simulink model "Energy_Cost"  (Simulink 8.8)
settings: Solver=ode23t  StartTime=0.0  StopTime=24  RelTol=1e-3  EnableMultiTasking=on
model workspace: external: MAT-File (data not in the file)
libraries: simulink x4
(part 4 of 5)

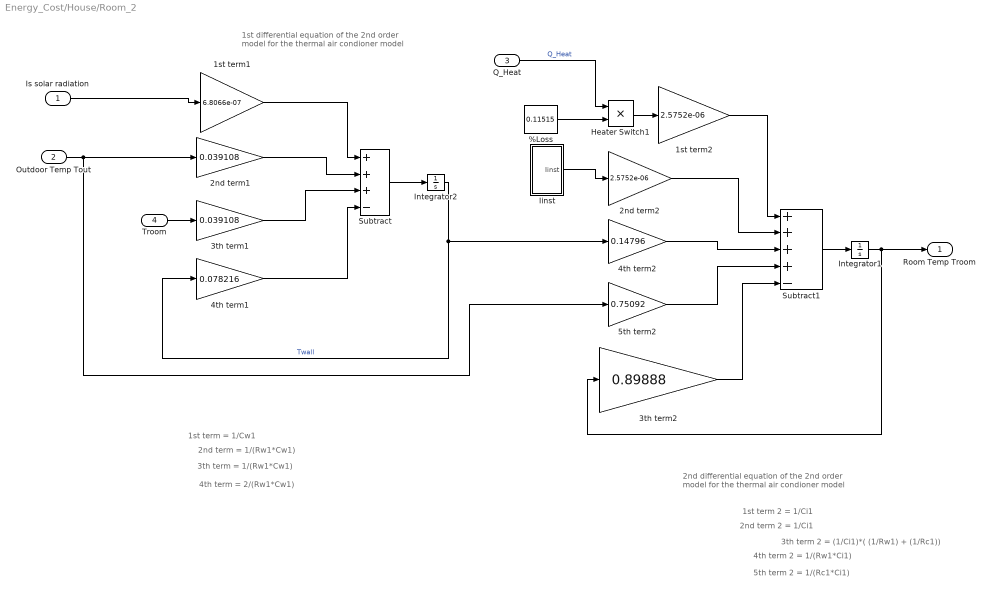
== system Energy_Cost/House/Room_2 ==
  note: 1st differential equation of the 2nd order
      | model for the thermal air condioner model
  note: 2nd differential equation of the 2nd order
      | model for the thermal air condioner model
  note: 1st term = 1/Cw1
  note: 2nd term = 1/(Rw1*Cw1)
  note: 3th term = 1/(Rw1*Cw1)
  note: 4th term = 2/(Rw1*Cw1)
  note: 1st term 2 = 1/Ci1
  note: 2nd term 2 = 1/Ci1
  note: 3th term 2 = (1/Ci1)*( (1/Rw1) + (1/Rc1))
  note: 4th term 2 = 1/(Rw1*Ci1)
  note: 5th term 2 = 1/(Rc1*Ci1)
  Is solar radiation : Inport
  Outdoor Temp Tout : Inport  Port=2
  Q_Heat : Inport  Port=3
  Troom : Inport  Port=4
  %Loss : Constant  Value=0.11515
  1st term1 : Gain  Gain=6.8066e-07
  1st term2 : Gain  Gain=2.5752e-06
  2nd term1 : Gain  Gain=0.039108
  2nd term2 : Gain  Gain=2.5752e-06
  3th term1 : Gain  Gain=0.039108
  3th term2 : Gain  Gain=0.89888
  4th term1 : Gain  Gain=0.078216
  4th term2 : Gain  Gain=0.14796
  5th term2 : Gain  Gain=0.75092
  Heater Switch1 : Product  RndMeth=Zero
  Iinst : Subsystem
  Integrator1 : Integrator  InitialCondition=21
  Integrator2 : Integrator  InitialCondition=21
  Subtract : Sum  Inputs=+++-
  Subtract1 : Sum  Inputs=++++-
  Room Temp Troom : Outport  InitialOutput=0
  wires:
  2nd term1/1 -> Subtract/2
  4th term1/1 -> Subtract/4
  Subtract/1 -> Integrator2/1
  Integrator2/1 -> 4th term1/1, 4th term2/1  "Twall"
  Integrator1/1 -> 3th term2/1, Room Temp Troom/1
  Subtract1/1 -> Integrator1/1
  Outdoor Temp Tout/1 -> 2nd term1/1, 5th term2/1
  Troom/1 -> 3th term1/1
  3th term1/1 -> Subtract/3
  1st term1/1 -> Subtract/1
  2nd term2/1 -> Subtract1/2
  Q_Heat/1 -> Heater Switch1/1  "Q_Heat"
  Iinst/1(Iinst) -> 2nd term2/1
  Is solar radiation/1 -> 1st term1/1
  4th term2/1 -> Subtract1/3
  5th term2/1 -> Subtract1/4
  3th term2/1 -> Subtract1/5
  %Loss/1 -> Heater Switch1/2
  Heater Switch1/1 -> 1st term2/1
  1st term2/1 -> Subtract1/1

== system Energy_Cost/House/Room_3 ==
  note: 1st differential equation of the 2nd order
      | model for the thermal air condioner model
  note: 2nd differential equation of the 2nd order
      | model for the thermal air condioner model
  note: 1st term = 1/Cw1
  note: 2nd term = 1/(Rw1*Cw1)
  note: 3th term = 1/(Rw1*Cw1)
  note: 4th term = 2/(Rw1*Cw1)
  note: 1st term 2 = 1/Ci1
  note: 2nd term 2 = 1/Ci1
  note: 3th term 2 = (1/Ci1)*( (1/Rw1) + (1/Rc1))
  note: 4th term 2 = 1/(Rw1*Ci1)
  note: 5th term 2 = 1/(Rc1*Ci1)
  Is solar radiation : Inport
  Outdoor Temp Tout : Inport  Port=2
  Q_Heat : Inport  Port=3
  Troom : Inport  Port=4
  %Loss : Constant  Value=0.11638
  1st term1 : Gain  Gain=6.0825e-07
  1st term2 : Gain  Gain=2.2533e-06
  2nd term1 : Gain  Gain=0.039108
  2nd term2 : Gain  Gain=2.2533e-06
  3th term1 : Gain  Gain=0.039108
  3th term2 : Gain  Gain=0.80194
  4th term1 : Gain  Gain=0.078216
  4th term2 : Gain  Gain=0.14488
  5th term2 : Gain  Gain=0.65706
  Heater Switch1 : Product  RndMeth=Zero
  Iinst : Subsystem
  Integrator1 : Integrator  InitialCondition=21
  Integrator2 : Integrator  InitialCondition=21
  Subtract : Sum  Inputs=+++-
  Subtract1 : Sum  Inputs=++++-
  Room Temp Troom : Outport  InitialOutput=0
  wires:
  2nd term1/1 -> Subtract/2
  4th term1/1 -> Subtract/4
  Subtract/1 -> Integrator2/1
  Integrator2/1 -> 4th term1/1, 4th term2/1  "Twall"
  Integrator1/1 -> 3th term2/1, Room Temp Troom/1
  Subtract1/1 -> Integrator1/1
  Outdoor Temp Tout/1 -> 2nd term1/1, 5th term2/1
  Troom/1 -> 3th term1/1
  3th term1/1 -> Subtract/3
  1st term1/1 -> Subtract/1
  2nd term2/1 -> Subtract1/2
  Q_Heat/1 -> Heater Switch1/1  "Q_Heat"
  Iinst/1(Iinst) -> 2nd term2/1
  Is solar radiation/1 -> 1st term1/1
  4th term2/1 -> Subtract1/3
  5th term2/1 -> Subtract1/4
  3th term2/1 -> Subtract1/5
  %Loss/1 -> Heater Switch1/2
  1st term2/1 -> Subtract1/1
  Heater Switch1/1 -> 1st term2/1

== system Energy_Cost/House/Room_4 ==
  note: 1st differential equation of the 2nd order
      | model for the thermal air condioner model
  note: 2nd differential equation of the 2nd order
      | model for the thermal air condioner model
  note: 1st term = 1/Cw1
  note: 2nd term = 1/(Rw1*Cw1)
  note: 3th term = 1/(Rw1*Cw1)
  note: 4th term = 2/(Rw1*Cw1)
  note: 1st term 2 = 1/Ci1
  note: 2nd term 2 = 1/Ci1
  note: 3th term 2 = (1/Ci1)*( (1/Rw1) + (1/Rc1))
  note: 4th term 2 = 1/(Rw1*Ci1)
  note: 5th term 2 = 1/(Rc1*Ci1)
  Is solar radiation : Inport
  Outdoor Temp Tout : Inport  Port=2
  Q_Heat : Inport  Port=3
  Troom : Inport  Port=4
  %Loss : Constant  Value=0.11393
  1st term1 : Gain  Gain=7.7264e-07
  1st term2 : Gain  Gain=3.0044e-06
  2nd term1 : Gain  Gain=0.039108
  2nd term2 : Gain  Gain=3.0044e-06
  3th term1 : Gain  Gain=0.039108
  3th term2 : Gain  Gain=1.0281
  4th term1 : Gain  Gain=0.078216
  4th term2 : Gain  Gain=0.15207
  5th term2 : Gain  Gain=0.87608
  Heater Switch1 : Product  RndMeth=Zero
  Iinst : Subsystem
  Integrator1 : Integrator  InitialCondition=21
  Integrator2 : Integrator  InitialCondition=21
  Subtract : Sum  Inputs=+++-
  Subtract1 : Sum  Inputs=++++-
  Room Temp Troom : Outport  InitialOutput=0
  wires:
  2nd term1/1 -> Subtract/2
  4th term1/1 -> Subtract/4
  Subtract/1 -> Integrator2/1
  Integrator2/1 -> 4th term1/1, 4th term2/1  "Twall"
  Integrator1/1 -> 3th term2/1, Room Temp Troom/1
  Subtract1/1 -> Integrator1/1
  Outdoor Temp Tout/1 -> 2nd term1/1, 5th term2/1
  Troom/1 -> 3th term1/1
  3th term1/1 -> Subtract/3
  1st term1/1 -> Subtract/1
  2nd term2/1 -> Subtract1/2
  Q_Heat/1 -> Heater Switch1/1  "Q_Heat"
  Iinst/1(Iinst) -> 2nd term2/1
  Is solar radiation/1 -> 1st term1/1
  4th term2/1 -> Subtract1/3
  5th term2/1 -> Subtract1/4
  3th term2/1 -> Subtract1/5
  %Loss/1 -> Heater Switch1/2
  Heater Switch1/1 -> 1st term2/1
  1st term2/1 -> Subtract1/1

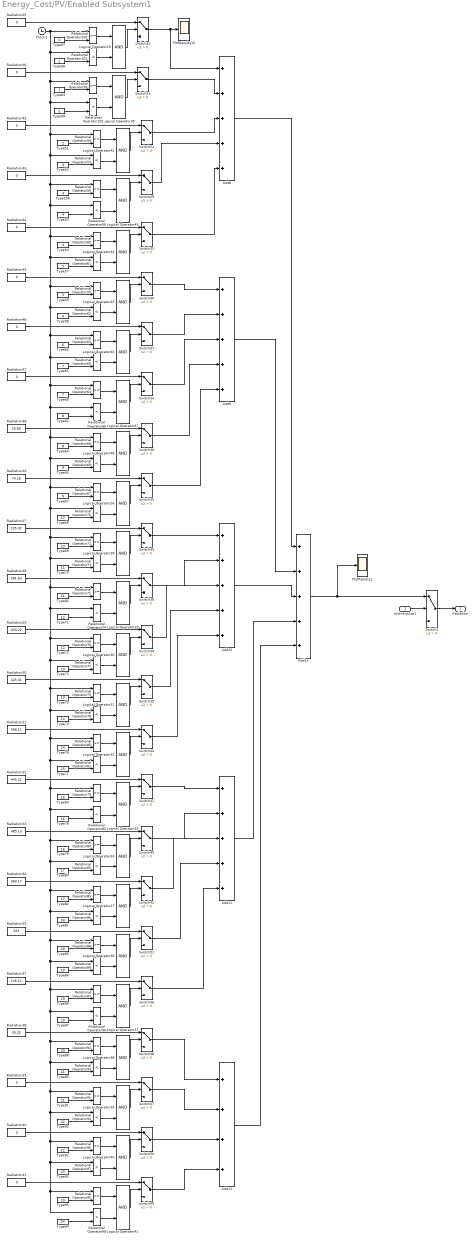
== system Energy_Cost/PV/Enabled Subsystem1 ==
  active pulse1 : Inport
  Add{8..11,13} (5 alike) : Sum  Inputs=+++++
  Add12 : Sum  Inputs=++++
  Clock2 : Clock
  Logical Operator{19,26..48} (24 alike) : Logic  AllPortsSameDT=off  OutDataTypeStr=boolean
  PlotResults1 : Scope
  PlotResults10 : Scope
  Radiation{25,36,39..47} (11 alike) : Constant  Value=0
  Radiation26 : Constant  Value=74.18
  Radiation27 : Constant  Value=195.32
  Radiation28 : Constant  Value=281.63
  Radiation29 : Constant  Value=453.22
  Radiation30 : Constant  Value=425.31
  Radiation31 : Constant  Value=556.11
  Radiation32 : Constant  Value=445.22
  Radiation33 : Constant  Value=485.13
  Radiation34 : Constant  Value=360.17
  Radiation35 : Constant  Value=253
  Radiation37 : Constant  Value=126.11
  Radiation38 : Constant  Value=33.25
  Radiation48 : Constant  Value=25.85
  Relational Operator{55..56,59..60,63..64,67..68,71..72,75..76,79..80,83..84,87..88,91..92,95..96,99..100} (24 alike) : RelationalOperator  RndMeth=Nearest  InputSameDT=on
  Relational Operator{57..58,61..62,65..66,69..70,73..74,77..78,81..82,85..86,89..90,93..94,97..98,101..102} (24 alike) : RelationalOperator  Operator=<  RndMeth=Nearest  InputSameDT=on
  Switch{1,29..30,33..54} (25 alike) : Switch  Criteria=u2 > Threshold
  Type100 : Constant  Value=3
  Type51 : Constant  Value=2
  Type52 : Constant  Value=3
  Type53 : Constant  Value=4
  Type54 : Constant  Value=4
  Type57 : Constant  Value=5
  Type58 : Constant  Value=6
  Type59 : Constant  Value=5
  Type60 : Constant  Value=6
  Type61 : Constant  Value=7
  Type62 : Constant  Value=8
  Type63 : Constant
  Type64 : Constant  Value=8
  Type65 : Constant  Value=9
  Type66 : Constant  Value=10
  Type67 : Constant  Value=9
  Type68 : Constant  Value=7
  Type69 : Constant  Value=10
  Type70 : Constant  Value=11
  Type71 : Constant  Value=12
  Type72 : Constant  Value=12
  Type73 : Constant  Value=13
  Type74 : Constant  Value=14
  Type75 : Constant  Value=13
  Type76 : Constant  Value=14
  Type77 : Constant  Value=15
  Type78 : Constant  Value=16
  Type79 : Constant  Value=16
  Type80 : Constant  Value=17
  Type81 : Constant  Value=18
  Type82 : Constant  Value=17
  Type83 : Constant  Value=15
  Type84 : Constant  Value=11
  Type85 : Constant  Value=18
  Type86 : Constant  Value=19
  Type87 : Constant  Value=20
  Type88 : Constant  Value=20
  Type89 : Constant  Value=21
  Type90 : Constant  Value=22
  Type91 : Constant  Value=21
  Type92 : Constant  Value=22
  Type93 : Constant  Value=23
  Type94 : Constant  Value=24
  Type95 : Constant  Value=23
  Type96 : Constant  Value=19
  Type97 : Constant  Value=0
  Type98 : Constant
  Type99 : Constant  Value=2
  Radiation : Outport
  wires:
  Switch1/1 -> Radiation/1
  active pulse1/1 -> Switch1/2
  Radiation25/1 -> Switch52/1
  Switch52/1 -> PlotResults10/1, Add8/1
  Clock2/1 -> Relational Operator100/1, Relational Operator101/1, Relational Operator99/1, Relational Operator102/1, Relational Operator64/1, Relational Operator65/1, Relational Operator63/1, Relational Operator66/1, Relational Operator68/1, Relational Operator69/1, Relational Operator67/1, Relational Operator70/1, Relational Operator72/1, Relational Operator73/1, Relational Operator71/1, Relational Operator76/1, Relational Operator75/1, Relational Operator78/1, Relational Operator80/1, Relational Operator81/1, Relational Operator79/1, Relational Operator82/1, Relational Operator84/1, Relational Operator85/1, Relational Operator83/1, Relational Operator86/1, Relational Operator89/1, Relational Operator87/1, Relational Operator91/1, Relational Operator98/1, Relational Operator95/1, Relational Operator97/1, Relational Operator96/1, Relational Operator94/1, Relational Operator93/1, Relational Operator92/1, Relational Operator90/1, Relational Operator88/1, Relational Operator77/1, Relational Operator74/1, Relational Operator62/1, Relational Operator59/1, Relational Operator61/1, Relational Operator60/1, Relational Operator58/1, Relational Operator55/1, Relational Operator57/1, Relational Operator56/1
  Type97/1 -> Relational Operator100/2
  Type98/1 -> Relational Operator101/2
  Relational Operator101/1 -> Logical Operator19/2
  Relational Operator100/1 -> Logical Operator19/1
  Logical Operator19/1 -> Switch52/2
  Radiation36/1 -> Switch53/1
  Type63/1 -> Relational Operator99/2
  Type99/1 -> Relational Operator102/2
  Relational Operator102/1 -> Logical Operator35/2
  Relational Operator99/1 -> Logical Operator35/1
  Logical Operator35/1 -> Switch53/2
  Type51/1 -> Relational Operator56/2
  Type52/1 -> Relational Operator57/2
  Relational Operator57/1 -> Logical Operator42/2
  Relational Operator56/1 -> Logical Operator42/1
  Logical Operator42/1 -> Switch54/2
  Type100/1 -> Relational Operator55/2
  Type53/1 -> Relational Operator58/2
  Relational Operator58/1 -> Logical Operator43/2
  Relational Operator55/1 -> Logical Operator43/1
  Logical Operator43/1 -> Switch29/2
  Type54/1 -> Relational Operator60/2
  Type57/1 -> Relational Operator61/2
  Relational Operator61/1 -> Logical Operator44/2
  Relational Operator60/1 -> Logical Operator44/1
  Logical Operator44/1 -> Switch33/2
  Type59/1 -> Relational Operator59/2
  Type58/1 -> Relational Operator62/2
  Relational Operator62/1 -> Logical Operator45/2
  Relational Operator59/1 -> Logical Operator45/1
  Logical Operator45/1 -> Switch30/2
  Type60/1 -> Relational Operator64/2
  Type61/1 -> Relational Operator65/2
  Relational Operator65/1 -> Logical Operator46/2
  Relational Operator64/1 -> Logical Operator46/1
  Logical Operator46/1 -> Switch37/2
  Type68/1 -> Relational Operator63/2
  Type62/1 -> Relational Operator66/2
  Relational Operator66/1 -> Logical Operator47/2
  Relational Operator63/1 -> Logical Operator47/1
  Logical Operator47/1 -> Switch34/2
  Type64/1 -> Relational Operator68/2
  Type65/1 -> Relational Operator69/2
  Relational Operator69/1 -> Logical Operator48/2
  Relational Operator68/1 -> Logical Operator48/1
  Logical Operator48/1 -> Switch36/2
  Type67/1 -> Relational Operator67/2
  Type66/1 -> Relational Operator70/2
  Relational Operator70/1 -> Logical Operator26/2
  Relational Operator67/1 -> Logical Operator26/1
  Logical Operator26/1 -> Switch35/2
  Type69/1 -> Relational Operator72/2
  Type70/1 -> Relational Operator73/2
  Relational Operator73/1 -> Logical Operator28/2
  Relational Operator72/1 -> Logical Operator28/1
  Logical Operator28/1 -> Switch45/2
  Type84/1 -> Relational Operator71/2
  Type71/1 -> Relational Operator74/2
  Relational Operator74/1 -> Logical Operator29/2
  Relational Operator71/1 -> Logical Operator29/1
  Logical Operator29/1 -> Switch38/2
  Type72/1 -> Relational Operator76/2
  Type73/1 -> Relational Operator77/2
  Relational Operator77/1 -> Logical Operator30/2
  Relational Operator76/1 -> Logical Operator30/1
  Logical Operator30/1 -> Switch40/2
  Type75/1 -> Relational Operator75/2
  Type74/1 -> Relational Operator78/2
  Relational Operator78/1 -> Logical Operator31/2
  Relational Operator75/1 -> Logical Operator31/1
  Logical Operator31/1 -> Switch39/2
  Type76/1 -> Relational Operator80/2
  Type77/1 -> Relational Operator81/2
  Relational Operator81/1 -> Logical Operator32/2
  Relational Operator80/1 -> Logical Operator32/1
  Logical Operator32/1 -> Switch44/2
  Type83/1 -> Relational Operator79/2
  Type78/1 -> Relational Operator82/2
  Relational Operator82/1 -> Logical Operator33/2
  Relational Operator79/1 -> Logical Operator33/1
  Logical Operator33/1 -> Switch41/2
  Type79/1 -> Relational Operator84/2
  Type80/1 -> Relational Operator85/2
  Relational Operator85/1 -> Logical Operator34/2
  Relational Operator84/1 -> Logical Operator34/1
  Logical Operator34/1 -> Switch43/2
  Type82/1 -> Relational Operator83/2
  Type81/1 -> Relational Operator86/2
  Relational Operator86/1 -> Logical Operator27/2
  Relational Operator83/1 -> Logical Operator27/1
  Logical Operator27/1 -> Switch42/2
  Type85/1 -> Relational Operator88/2
  Type86/1 -> Relational Operator89/2
  Relational Operator89/1 -> Logical Operator36/2
  Relational Operator88/1 -> Logical Operator36/1
  Logical Operator36/1 -> Switch51/2
  Type96/1 -> Relational Operator87/2
  Type87/1 -> Relational Operator90/2
  Relational Operator90/1 -> Logical Operator37/2
  Relational Operator87/1 -> Logical Operator37/1
  Logical Operator37/1 -> Switch46/2
  Type88/1 -> Relational Operator92/2
  Type89/1 -> Relational Operator93/2
  Relational Operator93/1 -> Logical Operator38/2
  Relational Operator92/1 -> Logical Operator38/1
  Logical Operator38/1 -> Switch48/2
  Type91/1 -> Relational Operator91/2
  Type90/1 -> Relational Operator94/2
  Relational Operator94/1 -> Logical Operator39/2
  Relational Operator91/1 -> Logical Operator39/1
  Logical Operator39/1 -> Switch47/2
  Type92/1 -> Relational Operator96/2
  Type93/1 -> Relational Operator97/2
  Relational Operator97/1 -> Logical Operator40/2
  Relational Operator96/1 -> Logical Operator40/1
  Logical Operator40/1 -> Switch50/2
  Type95/1 -> Relational Operator95/2
  Type94/1 -> Relational Operator98/2
  Relational Operator98/1 -> Logical Operator41/2
  Relational Operator95/1 -> Logical Operator41/1
  Logical Operator41/1 -> Switch49/2
  Radiation42/1 -> Switch54/1
  Radiation43/1 -> Switch29/1
  Radiation44/1 -> Switch33/1
  Radiation45/1 -> Switch30/1
  Radiation46/1 -> Switch37/1
  Radiation47/1 -> Switch34/1
  Radiation48/1 -> Switch36/1
  Radiation26/1 -> Switch35/1
  Radiation27/1 -> Switch45/1
  Radiation28/1 -> Switch38/1
  Radiation29/1 -> Switch40/1
  Radiation30/1 -> Switch39/1
  Radiation31/1 -> Switch44/1
  Radiation32/1 -> Switch41/1
  Radiation33/1 -> Switch43/1
  Radiation34/1 -> Switch42/1
  Radiation35/1 -> Switch51/1
  Radiation37/1 -> Switch46/1
  Radiation38/1 -> Switch48/1
  Radiation39/1 -> Switch47/1
  Radiation40/1 -> Switch50/1
  Radiation41/1 -> Switch49/1
  Switch53/1 -> Add8/2
  Switch54/1 -> Add8/3
  Switch33/1 -> Add8/5
  Switch29/1 -> Add8/4
  Switch30/1 -> Add9/1
  Switch37/1 -> Add9/2
  Switch34/1 -> Add9/3
  Switch36/1 -> Add9/4
  Switch35/1 -> Add9/5
  Switch45/1 -> Add10/1
  Switch38/1 -> Add10/2
  Switch40/1 -> Add10/3
  Switch39/1 -> Add10/4
  Switch44/1 -> Add10/5
  Switch41/1 -> Add11/1
  Switch43/1 -> Add11/2
  Switch42/1 -> Add11/3
  Switch51/1 -> Add11/4
  Switch46/1 -> Add11/5
  Switch48/1 -> Add12/1
  Switch47/1 -> Add12/2
  Switch50/1 -> Add12/3
  Switch49/1 -> Add12/4
  Add8/1 -> Add13/1
  Add9/1 -> Add13/2
  Add10/1 -> Add13/3
  Add11/1 -> Add13/4
  Add12/1 -> Add13/5
  Add13/1 -> Switch1/1, PlotResults1/1

== system Energy_Cost/PV/Rates ==
  Powe_cons : Inport
  Rate_season2 : Inport  Port=2
  Clock1 : Clock
      settings: Decimation=100
  Constant : Constant  Value=6.2
  Constant1 : Constant  Value=10.8
  Constant2 : Constant  Value=9.2
  Electricity Rate : M-S-Function  FunctionName=Elec_Rate_Fun
  Heater Switch1 : Product  RndMeth=Zero
  Rate : Outport  InitialOutput=0
  wires:
  Powe_cons/1 -> Heater Switch1/2
  Heater Switch1/1 -> Rate/1
  Constant/1 -> Electricity Rate/1
  Clock1/1 -> Electricity Rate/4
  Rate_season2/1 -> Electricity Rate/5
  Electricity Rate/1 -> Heater Switch1/1  "Elec_Rate"
  Constant2/1 -> Electricity Rate/2
  Constant1/1 -> Electricity Rate/3

== system Energy_Cost/Refrigerator/Rates ==
  Powe_cons : Inport
  Rate_season2 : Inport  Port=2
  Clock2 : Clock
      settings: Decimation=100
  Ele_mid : Constant  Value=9.2
  Ele_off : Constant  Value=6.2
  Ele_peak : Constant  Value=10.8
  Electricity Rate : M-S-Function  FunctionName=Elec_Rate_Fun
  Heater Switch6 : Product  Inputs=3  RndMeth=Zero
  Rate_Ele_WH : Constant
  Rate : Outport  InitialOutput=0
  wires:
  Ele_off/1 -> Electricity Rate/1
  Ele_mid/1 -> Electricity Rate/2
  Ele_peak/1 -> Electricity Rate/3
  Clock2/1 -> Electricity Rate/4
  Rate_Ele_WH/1 -> Heater Switch6/1
  Heater Switch6/1 -> Rate/1
  Powe_cons/1 -> Heater Switch6/3
  Rate_season2/1 -> Electricity Rate/5
  Electricity Rate/1 -> Heater Switch6/2

== system Energy_Cost/Thermostat/If Action Subsystem ==
  In1 : Inport
  Action Port : ActionPort  ActionType=then
  Out1 : Outport
  wires:
  In1/1 -> Out1/1

== system Energy_Cost/Thermostat/If Action Subsystem1 ==
  In1 : Inport
  Action Port : ActionPort  ActionType=else
  Out1 : Outport
  wires:
  In1/1 -> Out1/1

== system Energy_Cost/Water Heater/Rates ==
  Powe_cons : Inport
  Clock2 : Clock
      settings: Decimation=100
  Constant : Constant
  Ele_mid : Constant  Value=9.2
  Ele_off : Constant  Value=6.2
  Ele_peak : Constant  Value=10.8
  Electricity Rate : M-S-Function  FunctionName=Elec_Rate_Fun
  Gas rate : Constant  Value=35.7
  Heater Switch2 : Product  Inputs=3  RndMeth=Zero
  Heater Switch6 : Product  Inputs=3  RndMeth=Zero
  Rate_Ele_WH : Constant  Value=0
  Rate_Gas_WH : Constant
  Rate_season : Constant
  Sum2 : Sum  SaturateOnIntegerOverflow=on  InputSameDT=on  OutDataTypeStr=Inherit: Same as first input
  c3=Watts/Pc : Gain  Gain=1/9.932  SaturateOnIntegerOverflow=on  OutDataTypeStr=Inherit: Same as input  ParamDataTypeStr=Inherit: Same as input
  Rate : Outport  InitialOutput=0
  Rate_season1 : Outport  Port=2  InitialOutput=0
  wires:
  Ele_off/1 -> Electricity Rate/1
  Ele_mid/1 -> Electricity Rate/2
  Ele_peak/1 -> Electricity Rate/3
  Clock2/1 -> Electricity Rate/4
  Rate_season/1 -> Electricity Rate/5, Rate_season1/1
  Rate_Ele_WH/1 -> Heater Switch6/1
  Powe_cons/1 -> c3=Watts/Pc/1, Heater Switch6/3
  c3=Watts/Pc/1 -> Heater Switch2/1
  Gas rate/1 -> Heater Switch2/2
  Rate_Gas_WH/1 -> Heater Switch2/3
  Heater Switch6/1 -> Sum2/1
  Heater Switch2/1 -> Sum2/2
  Sum2/1 -> Rate/1
  Electricity Rate/1 -> Heater Switch6/2

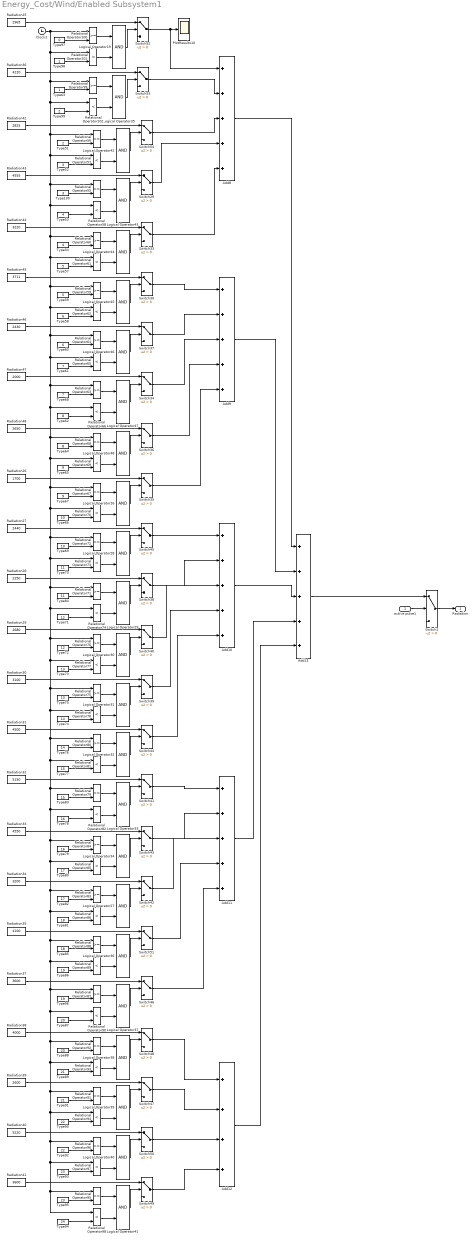
== system Energy_Cost/Wind/Enabled Subsystem1 ==
  active pulse1 : Inport
  Add{8..11,13} (5 alike) : Sum  Inputs=+++++
  Add12 : Sum  Inputs=++++
  Clock2 : Clock
  Logical Operator{19,26..48} (24 alike) : Logic  AllPortsSameDT=off  OutDataTypeStr=boolean
  PlotResults10 : Scope
  Radiation25 : Constant  Value=2965
  Radiation26 : Constant  Value=1700
  Radiation27 : Constant  Value=2440
  Radiation28 : Constant  Value=2250
  Radiation29 : Constant  Value=2680
  Radiation30 : Constant  Value=3100
  Radiation31 : Constant  Value=4500
  Radiation32 : Constant  Value=5150
  Radiation33 : Constant  Value=4550
  Radiation34 : Constant  Value=3200
  Radiation35 : Constant  Value=4100
  Radiation36 : Constant  Value=4220
  Radiation37 : Constant  Value=3600
  Radiation38 : Constant  Value=4000
  Radiation39 : Constant  Value=2600
  Radiation40 : Constant  Value=5220
  Radiation41 : Constant  Value=3600
  Radiation42 : Constant  Value=2825
  Radiation43 : Constant  Value=4555
  Radiation44 : Constant  Value=3220
  Radiation45 : Constant  Value=3711
  Radiation46 : Constant  Value=2430
  Radiation47 : Constant  Value=2000
  Radiation48 : Constant  Value=2650
  Relational Operator{55..56,59..60,63..64,67..68,71..72,75..76,79..80,83..84,87..88,91..92,95..96,99..100} (24 alike) : RelationalOperator  RndMeth=Nearest  InputSameDT=on
  Relational Operator{57..58,61..62,65..66,69..70,73..74,77..78,81..82,85..86,89..90,93..94,97..98,101..102} (24 alike) : RelationalOperator  Operator=<  RndMeth=Nearest  InputSameDT=on
  Switch{1,29..30,33..54} (25 alike) : Switch  Criteria=u2 > Threshold
  Type100 : Constant  Value=3
  Type51 : Constant  Value=2
  Type52 : Constant  Value=3
  Type53 : Constant  Value=4
  Type54 : Constant  Value=4
  Type57 : Constant  Value=5
  Type58 : Constant  Value=6
  Type59 : Constant  Value=5
  Type60 : Constant  Value=6
  Type61 : Constant  Value=7
  Type62 : Constant  Value=8
  Type63 : Constant
  Type64 : Constant  Value=8
  Type65 : Constant  Value=9
  Type66 : Constant  Value=10
  Type67 : Constant  Value=9
  Type68 : Constant  Value=7
  Type69 : Constant  Value=10
  Type70 : Constant  Value=11
  Type71 : Constant  Value=12
  Type72 : Constant  Value=12
  Type73 : Constant  Value=13
  Type74 : Constant  Value=14
  Type75 : Constant  Value=13
  Type76 : Constant  Value=14
  Type77 : Constant  Value=15
  Type78 : Constant  Value=16
  Type79 : Constant  Value=16
  Type80 : Constant  Value=17
  Type81 : Constant  Value=18
  Type82 : Constant  Value=17
  Type83 : Constant  Value=15
  Type84 : Constant  Value=11
  Type85 : Constant  Value=18
  Type86 : Constant  Value=19
  Type87 : Constant  Value=20
  Type88 : Constant  Value=20
  Type89 : Constant  Value=21
  Type90 : Constant  Value=22
  Type91 : Constant  Value=21
  Type92 : Constant  Value=22
  Type93 : Constant  Value=23
  Type94 : Constant  Value=24
  Type95 : Constant  Value=23
  Type96 : Constant  Value=19
  Type97 : Constant  Value=0
  Type98 : Constant
  Type99 : Constant  Value=2
  Radiation : Outport
  wires:
  Switch1/1 -> Radiation/1
  active pulse1/1 -> Switch1/2
  Radiation25/1 -> Switch52/1
  Switch52/1 -> PlotResults10/1, Add8/1
  Clock2/1 -> Relational Operator100/1, Relational Operator101/1, Relational Operator99/1, Relational Operator102/1, Relational Operator64/1, Relational Operator65/1, Relational Operator63/1, Relational Operator66/1, Relational Operator68/1, Relational Operator69/1, Relational Operator67/1, Relational Operator70/1, Relational Operator72/1, Relational Operator73/1, Relational Operator71/1, Relational Operator76/1, Relational Operator75/1, Relational Operator78/1, Relational Operator80/1, Relational Operator81/1, Relational Operator79/1, Relational Operator82/1, Relational Operator84/1, Relational Operator85/1, Relational Operator83/1, Relational Operator86/1, Relational Operator89/1, Relational Operator87/1, Relational Operator91/1, Relational Operator98/1, Relational Operator95/1, Relational Operator97/1, Relational Operator96/1, Relational Operator94/1, Relational Operator93/1, Relational Operator92/1, Relational Operator90/1, Relational Operator88/1, Relational Operator77/1, Relational Operator74/1, Relational Operator62/1, Relational Operator59/1, Relational Operator61/1, Relational Operator60/1, Relational Operator58/1, Relational Operator55/1, Relational Operator57/1, Relational Operator56/1
  Type97/1 -> Relational Operator100/2
  Type98/1 -> Relational Operator101/2
  Relational Operator101/1 -> Logical Operator19/2
  Relational Operator100/1 -> Logical Operator19/1
  Logical Operator19/1 -> Switch52/2
  Radiation36/1 -> Switch53/1
  Type63/1 -> Relational Operator99/2
  Type99/1 -> Relational Operator102/2
  Relational Operator102/1 -> Logical Operator35/2
  Relational Operator99/1 -> Logical Operator35/1
  Logical Operator35/1 -> Switch53/2
  Type51/1 -> Relational Operator56/2
  Type52/1 -> Relational Operator57/2
  Relational Operator57/1 -> Logical Operator42/2
  Relational Operator56/1 -> Logical Operator42/1
  Logical Operator42/1 -> Switch54/2
  Type100/1 -> Relational Operator55/2
  Type53/1 -> Relational Operator58/2
  Relational Operator58/1 -> Logical Operator43/2
  Relational Operator55/1 -> Logical Operator43/1
  Logical Operator43/1 -> Switch29/2
  Type54/1 -> Relational Operator60/2
  Type57/1 -> Relational Operator61/2
  Relational Operator61/1 -> Logical Operator44/2
  Relational Operator60/1 -> Logical Operator44/1
  Logical Operator44/1 -> Switch33/2
  Type59/1 -> Relational Operator59/2
  Type58/1 -> Relational Operator62/2
  Relational Operator62/1 -> Logical Operator45/2
  Relational Operator59/1 -> Logical Operator45/1
  Logical Operator45/1 -> Switch30/2
  Type60/1 -> Relational Operator64/2
  Type61/1 -> Relational Operator65/2
  Relational Operator65/1 -> Logical Operator46/2
  Relational Operator64/1 -> Logical Operator46/1
  Logical Operator46/1 -> Switch37/2
  Type68/1 -> Relational Operator63/2
  Type62/1 -> Relational Operator66/2
  Relational Operator66/1 -> Logical Operator47/2
  Relational Operator63/1 -> Logical Operator47/1
  Logical Operator47/1 -> Switch34/2
  Type64/1 -> Relational Operator68/2
  Type65/1 -> Relational Operator69/2
  Relational Operator69/1 -> Logical Operator48/2
  Relational Operator68/1 -> Logical Operator48/1
  Logical Operator48/1 -> Switch36/2
  Type67/1 -> Relational Operator67/2
  Type66/1 -> Relational Operator70/2
  Relational Operator70/1 -> Logical Operator26/2
  Relational Operator67/1 -> Logical Operator26/1
  Logical Operator26/1 -> Switch35/2
  Type69/1 -> Relational Operator72/2
  Type70/1 -> Relational Operator73/2
  Relational Operator73/1 -> Logical Operator28/2
  Relational Operator72/1 -> Logical Operator28/1
  Logical Operator28/1 -> Switch45/2
  Type84/1 -> Relational Operator71/2
  Type71/1 -> Relational Operator74/2
  Relational Operator74/1 -> Logical Operator29/2
  Relational Operator71/1 -> Logical Operator29/1
  Logical Operator29/1 -> Switch38/2
  Type72/1 -> Relational Operator76/2
  Type73/1 -> Relational Operator77/2
  Relational Operator77/1 -> Logical Operator30/2
  Relational Operator76/1 -> Logical Operator30/1
  Logical Operator30/1 -> Switch40/2
  Type75/1 -> Relational Operator75/2
  Type74/1 -> Relational Operator78/2
  Relational Operator78/1 -> Logical Operator31/2
  Relational Operator75/1 -> Logical Operator31/1
  Logical Operator31/1 -> Switch39/2
  Type76/1 -> Relational Operator80/2
  Type77/1 -> Relational Operator81/2
  Relational Operator81/1 -> Logical Operator32/2
  Relational Operator80/1 -> Logical Operator32/1
  Logical Operator32/1 -> Switch44/2
  Type83/1 -> Relational Operator79/2
  Type78/1 -> Relational Operator82/2
  Relational Operator82/1 -> Logical Operator33/2
  Relational Operator79/1 -> Logical Operator33/1
  Logical Operator33/1 -> Switch41/2
  Type79/1 -> Relational Operator84/2
  Type80/1 -> Relational Operator85/2
  Relational Operator85/1 -> Logical Operator34/2
  Relational Operator84/1 -> Logical Operator34/1
  Logical Operator34/1 -> Switch43/2
  Type82/1 -> Relational Operator83/2
  Type81/1 -> Relational Operator86/2
  Relational Operator86/1 -> Logical Operator27/2
  Relational Operator83/1 -> Logical Operator27/1
  Logical Operator27/1 -> Switch42/2
  Type85/1 -> Relational Operator88/2
  Type86/1 -> Relational Operator89/2
  Relational Operator89/1 -> Logical Operator36/2
  Relational Operator88/1 -> Logical Operator36/1
  Logical Operator36/1 -> Switch51/2
  Type96/1 -> Relational Operator87/2
  Type87/1 -> Relational Operator90/2
  Relational Operator90/1 -> Logical Operator37/2
  Relational Operator87/1 -> Logical Operator37/1
  Logical Operator37/1 -> Switch46/2
  Type88/1 -> Relational Operator92/2
  Type89/1 -> Relational Operator93/2
  Relational Operator93/1 -> Logical Operator38/2
  Relational Operator92/1 -> Logical Operator38/1
  Logical Operator38/1 -> Switch48/2
  Type91/1 -> Relational Operator91/2
  Type90/1 -> Relational Operator94/2
  Relational Operator94/1 -> Logical Operator39/2
  Relational Operator91/1 -> Logical Operator39/1
  Logical Operator39/1 -> Switch47/2
  Type92/1 -> Relational Operator96/2
  Type93/1 -> Relational Operator97/2
  Relational Operator97/1 -> Logical Operator40/2
  Relational Operator96/1 -> Logical Operator40/1
  Logical Operator40/1 -> Switch50/2
  Type95/1 -> Relational Operator95/2
  Type94/1 -> Relational Operator98/2
  Relational Operator98/1 -> Logical Operator41/2
  Relational Operator95/1 -> Logical Operator41/1
  Logical Operator41/1 -> Switch49/2
  Radiation42/1 -> Switch54/1
  Radiation43/1 -> Switch29/1
  Radiation44/1 -> Switch33/1
  Radiation45/1 -> Switch30/1
  Radiation46/1 -> Switch37/1
  Radiation47/1 -> Switch34/1
  Radiation48/1 -> Switch36/1
  Radiation26/1 -> Switch35/1
  Radiation27/1 -> Switch45/1
  Radiation28/1 -> Switch38/1
  Radiation29/1 -> Switch40/1
  Radiation30/1 -> Switch39/1
  Radiation31/1 -> Switch44/1
  Radiation32/1 -> Switch41/1
  Radiation33/1 -> Switch43/1
  Radiation34/1 -> Switch42/1
  Radiation35/1 -> Switch51/1
  Radiation37/1 -> Switch46/1
  Radiation38/1 -> Switch48/1
  Radiation39/1 -> Switch47/1
  Radiation40/1 -> Switch50/1
  Radiation41/1 -> Switch49/1
  Switch53/1 -> Add8/2
  Switch54/1 -> Add8/3
  Switch33/1 -> Add8/5
  Switch29/1 -> Add8/4
  Switch30/1 -> Add9/1
  Switch37/1 -> Add9/2
  Switch34/1 -> Add9/3
  Switch36/1 -> Add9/4
  Switch35/1 -> Add9/5
  Switch45/1 -> Add10/1
  Switch38/1 -> Add10/2
  Switch40/1 -> Add10/3
  Switch39/1 -> Add10/4
  Switch44/1 -> Add10/5
  Switch41/1 -> Add11/1
  Switch43/1 -> Add11/2
  Switch42/1 -> Add11/3
  Switch51/1 -> Add11/4
  Switch46/1 -> Add11/5
  Switch48/1 -> Add12/1
  Switch47/1 -> Add12/2
  Switch50/1 -> Add12/3
  Switch49/1 -> Add12/4
  Add8/1 -> Add13/1
  Add9/1 -> Add13/2
  Add10/1 -> Add13/3
  Add11/1 -> Add13/4
  Add12/1 -> Add13/5
  Add13/1 -> Switch1/1

== system Energy_Cost/Wind/Rates ==
  Powe_cons : Inport
  Rate_season2 : Inport  Port=2
  Clock1 : Clock
      settings: Decimation=100
  Constant : Constant  Value=6.2
  Constant1 : Constant  Value=10.8
  Constant2 : Constant  Value=9.2
  Electricity Rate : M-S-Function  FunctionName=Elec_Rate_Fun
  Heater Switch1 : Product  RndMeth=Zero
  Rate : Outport  InitialOutput=0
  wires:
  Powe_cons/1 -> Heater Switch1/2
  Heater Switch1/1 -> Rate/1
  Constant/1 -> Electricity Rate/1
  Clock1/1 -> Electricity Rate/4
  Rate_season2/1 -> Electricity Rate/5
  Electricity Rate/1 -> Heater Switch1/1  "Elec_Rate"
  Constant1/1 -> Electricity Rate/3
  Constant2/1 -> Electricity Rate/2

== system Energy_Cost/Air Conditioner/Cost_AA/Rates ==
  Powe_cons : Inport
  Rate_season2 : Inport  Port=2
  Clock1 : Clock
      settings: Decimation=100
  Constant : Constant  Value=6.2
  Constant1 : Constant  Value=9.2
  Constant2 : Constant  Value=10.8
  Electricity Rate : M-S-Function  FunctionName=Elec_Rate_Fun
  Gas rate : Constant  Value=35.7
  Heater Switch2 : Product  Inputs=3  RndMeth=Zero
  Heater Switch6 : Product  Inputs=3  RndMeth=Zero
  Rate_Ele_WH : Constant  Value=0
  Rate_Gas_WH : Constant
  Sum2 : Sum  SaturateOnIntegerOverflow=on  InputSameDT=on  OutDataTypeStr=Inherit: Same as first input
  c3=Watts/Pc : Gain  Gain=1/9.932  SaturateOnIntegerOverflow=on  OutDataTypeStr=Inherit: Same as input  ParamDataTypeStr=Inherit: Same as input
  Rate : Outport  InitialOutput=0
  wires:
  Constant/1 -> Electricity Rate/1
  Constant1/1 -> Electricity Rate/2
  Constant2/1 -> Electricity Rate/3
  Clock1/1 -> Electricity Rate/4
  Rate_season2/1 -> Electricity Rate/5
  Rate_Ele_WH/1 -> Heater Switch6/1
  Powe_cons/1 -> c3=Watts/Pc/1, Heater Switch6/3
  c3=Watts/Pc/1 -> Heater Switch2/1
  Gas rate/1 -> Heater Switch2/2
  Rate_Gas_WH/1 -> Heater Switch2/3
  Heater Switch6/1 -> Sum2/1
  Heater Switch2/1 -> Sum2/2
  Sum2/1 -> Rate/1
  Electricity Rate/1 -> Heater Switch6/2  "Elec_Rate"

== system Energy_Cost/Battery/Enabled Subsystem1/Subsystem ==
  In1 : Inport
  In2 : Inport  Port=2
  Clock2 : Clock
  Divide26 : Product  Inputs=*/
  Dot Product2 : DotProduct  InputSameDT=on  OutDataTypeStr=Inherit: Inherit via internal rule
  Logical Operator19 : Logic  AllPortsSameDT=off  OutDataTypeStr=boolean
  Relational Operator2 : RelationalOperator  RndMeth=Nearest  InputSameDT=on
  Relational Operator3 : RelationalOperator  Operator=<  RndMeth=Nearest  InputSameDT=on
  Sum : Sum  Inputs=|++
  Sum1 : Sum  Inputs=|-+
  Switch2 : Switch  Criteria=u2 > Threshold
  Type54 : Constant
  Type57 : Constant  Value=0
  Type58 : Constant
  soc3 : Scope
  Out1 : Outport
  wires:
  Sum1/1 -> Divide26/1
  Type54/1 -> Divide26/2
  Divide26/1 -> Dot Product2/1
  Clock2/1 -> Dot Product2/2, Relational Operator3/1, Relational Operator2/1
  Dot Product2/1 -> Sum/2
  Sum/1 -> Switch2/1
  Type57/1 -> Relational Operator2/2
  Relational Operator2/1 -> Logical Operator19/1
  Type58/1 -> Relational Operator3/2
  Relational Operator3/1 -> Logical Operator19/2
  Logical Operator19/1 -> Switch2/2
  In1/1 -> Sum/1, Sum1/1
  In2/1 -> Sum1/2
  Switch2/1 -> Out1/1, soc3/1

== system Energy_Cost/Battery/Enabled Subsystem1/Subsystem1 ==
  In1 : Inport
  In2 : Inport  Port=2
  Clock2 : Clock
  Divide26 : Product  Inputs=*/
  Dot Product2 : DotProduct  InputSameDT=on  OutDataTypeStr=Inherit: Inherit via internal rule
  Logical Operator19 : Logic  AllPortsSameDT=off  OutDataTypeStr=boolean
  Relational Operator2 : RelationalOperator  RndMeth=Nearest  InputSameDT=on
  Relational Operator3 : RelationalOperator  Operator=<  RndMeth=Nearest  InputSameDT=on
  Sum : Sum  Inputs=|++
  Sum1 : Sum  Inputs=|-+
  Sum2 : Sum  Inputs=|+-
  Switch2 : Switch  Criteria=u2 > Threshold
  Type1 : Constant
  Type54 : Constant
  Type57 : Constant
  Type58 : Constant  Value=2
  soc1 : Scope
  Out1 : Outport
  wires:
  Switch2/1 -> Out1/1, soc1/1
  In2/1 -> Sum1/2
  In1/1 -> Sum1/1, Sum/1
  Logical Operator19/1 -> Switch2/2
  Relational Operator3/1 -> Logical Operator19/2
  Type58/1 -> Relational Operator3/2
  Relational Operator2/1 -> Logical Operator19/1
  Type57/1 -> Relational Operator2/2
  Sum/1 -> Switch2/1
  Dot Product2/1 -> Sum/2
  Divide26/1 -> Dot Product2/1
  Type54/1 -> Divide26/2
  Sum1/1 -> Divide26/1
  Clock2/1 -> Sum2/1, Relational Operator2/1, Relational Operator3/1
  Type1/1 -> Sum2/2
  Sum2/1 -> Dot Product2/2

== system Energy_Cost/Battery/Enabled Subsystem1/Subsystem10 ==
  In1 : Inport
  In2 : Inport  Port=2
  Clock2 : Clock
  Divide26 : Product  Inputs=*/
  Dot Product2 : DotProduct  InputSameDT=on  OutDataTypeStr=Inherit: Inherit via internal rule
  Logical Operator19 : Logic  AllPortsSameDT=off  OutDataTypeStr=boolean
  Relational Operator2 : RelationalOperator  RndMeth=Nearest  InputSameDT=on
  Relational Operator3 : RelationalOperator  Operator=<  RndMeth=Nearest  InputSameDT=on
  Sum : Sum  Inputs=|++
  Sum1 : Sum  Inputs=|-+
  Sum2 : Sum  Inputs=|+-
  Switch2 : Switch  Criteria=u2 > Threshold
  Type1 : Constant  Value=10
  Type54 : Constant
  Type57 : Constant  Value=10
  Type58 : Constant  Value=11
  soc1 : Scope
  Out1 : Outport
  wires:
  Sum2/1 -> Dot Product2/2
  Type1/1 -> Sum2/2
  Clock2/1 -> Relational Operator3/1, Relational Operator2/1, Sum2/1
  Sum1/1 -> Divide26/1
  Type54/1 -> Divide26/2
  Divide26/1 -> Dot Product2/1
  Dot Product2/1 -> Sum/2
  Sum/1 -> Switch2/1
  Type57/1 -> Relational Operator2/2
  Relational Operator2/1 -> Logical Operator19/1
  Type58/1 -> Relational Operator3/2
  Relational Operator3/1 -> Logical Operator19/2
  Logical Operator19/1 -> Switch2/2
  In1/1 -> Sum/1, Sum1/1
  In2/1 -> Sum1/2
  Switch2/1 -> soc1/1, Out1/1

== system Energy_Cost/Battery/Enabled Subsystem1/Subsystem11 ==
  In1 : Inport
  In2 : Inport  Port=2
  Clock2 : Clock
  Divide26 : Product  Inputs=*/
  Dot Product2 : DotProduct  InputSameDT=on  OutDataTypeStr=Inherit: Inherit via internal rule
  Logical Operator19 : Logic  AllPortsSameDT=off  OutDataTypeStr=boolean
  Relational Operator2 : RelationalOperator  RndMeth=Nearest  InputSameDT=on
  Relational Operator3 : RelationalOperator  Operator=<  RndMeth=Nearest  InputSameDT=on
  Sum : Sum  Inputs=|++
  Sum1 : Sum  Inputs=|-+
  Sum2 : Sum  Inputs=|+-
  Switch2 : Switch  Criteria=u2 > Threshold
  Type1 : Constant  Value=11
  Type54 : Constant
  Type57 : Constant  Value=11
  Type58 : Constant  Value=12
  soc1 : Scope
  Out1 : Outport
  wires:
  Switch2/1 -> Out1/1, soc1/1
  In2/1 -> Sum1/2
  In1/1 -> Sum1/1, Sum/1
  Logical Operator19/1 -> Switch2/2
  Relational Operator3/1 -> Logical Operator19/2
  Type58/1 -> Relational Operator3/2
  Relational Operator2/1 -> Logical Operator19/1
  Type57/1 -> Relational Operator2/2
  Sum/1 -> Switch2/1
  Dot Product2/1 -> Sum/2
  Divide26/1 -> Dot Product2/1
  Type54/1 -> Divide26/2
  Sum1/1 -> Divide26/1
  Clock2/1 -> Sum2/1, Relational Operator2/1, Relational Operator3/1
  Type1/1 -> Sum2/2
  Sum2/1 -> Dot Product2/2

== system Energy_Cost/Battery/Enabled Subsystem1/Subsystem12 ==
  In1 : Inport
  In2 : Inport  Port=2
  Clock2 : Clock
  Divide26 : Product  Inputs=*/
  Dot Product2 : DotProduct  InputSameDT=on  OutDataTypeStr=Inherit: Inherit via internal rule
  Logical Operator19 : Logic  AllPortsSameDT=off  OutDataTypeStr=boolean
  Relational Operator2 : RelationalOperator  RndMeth=Nearest  InputSameDT=on
  Relational Operator3 : RelationalOperator  Operator=<  RndMeth=Nearest  InputSameDT=on
  Sum : Sum  Inputs=|++
  Sum1 : Sum  Inputs=|-+
  Sum2 : Sum  Inputs=|+-
  Switch2 : Switch  Criteria=u2 > Threshold
  Type1 : Constant  Value=12
  Type54 : Constant
  Type57 : Constant  Value=12
  Type58 : Constant  Value=13
  soc1 : Scope
  Out1 : Outport
  wires:
  Sum2/1 -> Dot Product2/2
  Type1/1 -> Sum2/2
  Clock2/1 -> Relational Operator3/1, Relational Operator2/1, Sum2/1
  Sum1/1 -> Divide26/1
  Type54/1 -> Divide26/2
  Divide26/1 -> Dot Product2/1
  Dot Product2/1 -> Sum/2
  Sum/1 -> Switch2/1
  Type57/1 -> Relational Operator2/2
  Relational Operator2/1 -> Logical Operator19/1
  Type58/1 -> Relational Operator3/2
  Relational Operator3/1 -> Logical Operator19/2
  Logical Operator19/1 -> Switch2/2
  In1/1 -> Sum/1, Sum1/1
  In2/1 -> Sum1/2
  Switch2/1 -> soc1/1, Out1/1

== system Energy_Cost/Battery/Enabled Subsystem1/Subsystem13 ==
  In1 : Inport
  In2 : Inport  Port=2
  Clock2 : Clock
  Divide26 : Product  Inputs=*/
  Dot Product2 : DotProduct  InputSameDT=on  OutDataTypeStr=Inherit: Inherit via internal rule
  Logical Operator19 : Logic  AllPortsSameDT=off  OutDataTypeStr=boolean
  Relational Operator2 : RelationalOperator  RndMeth=Nearest  InputSameDT=on
  Relational Operator3 : RelationalOperator  Operator=<  RndMeth=Nearest  InputSameDT=on
  Sum : Sum  Inputs=|++
  Sum1 : Sum  Inputs=|-+
  Sum2 : Sum  Inputs=|+-
  Switch2 : Switch  Criteria=u2 > Threshold
  Type1 : Constant  Value=13
  Type54 : Constant
  Type57 : Constant  Value=13
  Type58 : Constant  Value=14
  soc1 : Scope
  Out1 : Outport
  wires:
  Switch2/1 -> Out1/1, soc1/1
  In2/1 -> Sum1/2
  In1/1 -> Sum1/1, Sum/1
  Logical Operator19/1 -> Switch2/2
  Relational Operator3/1 -> Logical Operator19/2
  Type58/1 -> Relational Operator3/2
  Relational Operator2/1 -> Logical Operator19/1
  Type57/1 -> Relational Operator2/2
  Sum/1 -> Switch2/1
  Dot Product2/1 -> Sum/2
  Divide26/1 -> Dot Product2/1
  Type54/1 -> Divide26/2
  Sum1/1 -> Divide26/1
  Clock2/1 -> Sum2/1, Relational Operator2/1, Relational Operator3/1
  Type1/1 -> Sum2/2
  Sum2/1 -> Dot Product2/2

== system Energy_Cost/Battery/Enabled Subsystem1/Subsystem14 ==
  In1 : Inport
  In2 : Inport  Port=2
  Clock2 : Clock
  Divide26 : Product  Inputs=*/
  Dot Product2 : DotProduct  InputSameDT=on  OutDataTypeStr=Inherit: Inherit via internal rule
  Logical Operator19 : Logic  AllPortsSameDT=off  OutDataTypeStr=boolean
  Relational Operator2 : RelationalOperator  RndMeth=Nearest  InputSameDT=on
  Relational Operator3 : RelationalOperator  Operator=<  RndMeth=Nearest  InputSameDT=on
  Sum : Sum  Inputs=|++
  Sum1 : Sum  Inputs=|-+
  Sum2 : Sum  Inputs=|+-
  Switch2 : Switch  Criteria=u2 > Threshold
  Type1 : Constant  Value=14
  Type54 : Constant
  Type57 : Constant  Value=14
  Type58 : Constant  Value=15
  soc1 : Scope
  Out1 : Outport
  wires:
  Sum2/1 -> Dot Product2/2
  Type1/1 -> Sum2/2
  Clock2/1 -> Relational Operator3/1, Relational Operator2/1, Sum2/1
  Sum1/1 -> Divide26/1
  Type54/1 -> Divide26/2
  Divide26/1 -> Dot Product2/1
  Dot Product2/1 -> Sum/2
  Sum/1 -> Switch2/1
  Type57/1 -> Relational Operator2/2
  Relational Operator2/1 -> Logical Operator19/1
  Type58/1 -> Relational Operator3/2
  Relational Operator3/1 -> Logical Operator19/2
  Logical Operator19/1 -> Switch2/2
  In1/1 -> Sum/1, Sum1/1
  In2/1 -> Sum1/2
  Switch2/1 -> soc1/1, Out1/1

== system Energy_Cost/Battery/Enabled Subsystem1/Subsystem15 ==
  In1 : Inport
  In2 : Inport  Port=2
  Clock2 : Clock
  Divide26 : Product  Inputs=*/
  Dot Product2 : DotProduct  InputSameDT=on  OutDataTypeStr=Inherit: Inherit via internal rule
  Logical Operator19 : Logic  AllPortsSameDT=off  OutDataTypeStr=boolean
  Relational Operator2 : RelationalOperator  RndMeth=Nearest  InputSameDT=on
  Relational Operator3 : RelationalOperator  Operator=<  RndMeth=Nearest  InputSameDT=on
  Sum : Sum  Inputs=|++
  Sum1 : Sum  Inputs=|-+
  Sum2 : Sum  Inputs=|+-
  Switch2 : Switch  Criteria=u2 > Threshold
  Type1 : Constant  Value=15
  Type54 : Constant
  Type57 : Constant  Value=15
  Type58 : Constant  Value=16
  soc1 : Scope
  Out1 : Outport
  wires:
  Switch2/1 -> Out1/1, soc1/1
  In2/1 -> Sum1/2
  In1/1 -> Sum1/1, Sum/1
  Logical Operator19/1 -> Switch2/2
  Relational Operator3/1 -> Logical Operator19/2
  Type58/1 -> Relational Operator3/2
  Relational Operator2/1 -> Logical Operator19/1
  Type57/1 -> Relational Operator2/2
  Sum/1 -> Switch2/1
  Dot Product2/1 -> Sum/2
  Divide26/1 -> Dot Product2/1
  Type54/1 -> Divide26/2
  Sum1/1 -> Divide26/1
  Clock2/1 -> Sum2/1, Relational Operator2/1, Relational Operator3/1
  Type1/1 -> Sum2/2
  Sum2/1 -> Dot Product2/2

== system Energy_Cost/Battery/Enabled Subsystem1/Subsystem16 ==
  In1 : Inport
  In2 : Inport  Port=2
  Clock2 : Clock
  Divide26 : Product  Inputs=*/
  Dot Product2 : DotProduct  InputSameDT=on  OutDataTypeStr=Inherit: Inherit via internal rule
  Logical Operator19 : Logic  AllPortsSameDT=off  OutDataTypeStr=boolean
  Relational Operator2 : RelationalOperator  RndMeth=Nearest  InputSameDT=on
  Relational Operator3 : RelationalOperator  Operator=<  RndMeth=Nearest  InputSameDT=on
  Sum : Sum  Inputs=|++
  Sum1 : Sum  Inputs=|-+
  Sum2 : Sum  Inputs=|+-
  Switch2 : Switch  Criteria=u2 > Threshold
  Type1 : Constant  Value=16
  Type54 : Constant
  Type57 : Constant  Value=16
  Type58 : Constant  Value=17
  soc1 : Scope
  Out1 : Outport
  wires:
  Sum2/1 -> Dot Product2/2
  Type1/1 -> Sum2/2
  Clock2/1 -> Relational Operator3/1, Relational Operator2/1, Sum2/1
  Sum1/1 -> Divide26/1
  Type54/1 -> Divide26/2
  Divide26/1 -> Dot Product2/1
  Dot Product2/1 -> Sum/2
  Sum/1 -> Switch2/1
  Type57/1 -> Relational Operator2/2
  Relational Operator2/1 -> Logical Operator19/1
  Type58/1 -> Relational Operator3/2
  Relational Operator3/1 -> Logical Operator19/2
  Logical Operator19/1 -> Switch2/2
  In1/1 -> Sum/1, Sum1/1
  In2/1 -> Sum1/2
  Switch2/1 -> soc1/1, Out1/1

== system Energy_Cost/Battery/Enabled Subsystem1/Subsystem17 ==
  In1 : Inport
  In2 : Inport  Port=2
  Clock2 : Clock
  Divide26 : Product  Inputs=*/
  Dot Product2 : DotProduct  InputSameDT=on  OutDataTypeStr=Inherit: Inherit via internal rule
  Logical Operator19 : Logic  AllPortsSameDT=off  OutDataTypeStr=boolean
  Relational Operator2 : RelationalOperator  RndMeth=Nearest  InputSameDT=on
  Relational Operator3 : RelationalOperator  Operator=<  RndMeth=Nearest  InputSameDT=on
  Sum : Sum  Inputs=|++
  Sum1 : Sum  Inputs=|-+
  Sum2 : Sum  Inputs=|+-
  Switch2 : Switch  Criteria=u2 > Threshold
  Type1 : Constant  Value=17
  Type54 : Constant
  Type57 : Constant  Value=17
  Type58 : Constant  Value=18
  soc1 : Scope
  Out1 : Outport
  wires:
  Sum2/1 -> Dot Product2/2
  Type1/1 -> Sum2/2
  Clock2/1 -> Relational Operator3/1, Relational Operator2/1, Sum2/1
  Sum1/1 -> Divide26/1
  Type54/1 -> Divide26/2
  Divide26/1 -> Dot Product2/1
  Dot Product2/1 -> Sum/2
  Sum/1 -> Switch2/1
  Type57/1 -> Relational Operator2/2
  Relational Operator2/1 -> Logical Operator19/1
  Type58/1 -> Relational Operator3/2
  Relational Operator3/1 -> Logical Operator19/2
  Logical Operator19/1 -> Switch2/2
  In1/1 -> Sum/1, Sum1/1
  In2/1 -> Sum1/2
  Switch2/1 -> soc1/1, Out1/1

== system Energy_Cost/Battery/Enabled Subsystem1/Subsystem18 ==
  In1 : Inport
  In2 : Inport  Port=2
  Clock2 : Clock
  Divide26 : Product  Inputs=*/
  Dot Product2 : DotProduct  InputSameDT=on  OutDataTypeStr=Inherit: Inherit via internal rule
  Logical Operator19 : Logic  AllPortsSameDT=off  OutDataTypeStr=boolean
  Relational Operator2 : RelationalOperator  RndMeth=Nearest  InputSameDT=on
  Relational Operator3 : RelationalOperator  Operator=<  RndMeth=Nearest  InputSameDT=on
  Sum : Sum  Inputs=|++
  Sum1 : Sum  Inputs=|-+
  Sum2 : Sum  Inputs=|+-
  Switch2 : Switch  Criteria=u2 > Threshold
  Type1 : Constant  Value=18
  Type54 : Constant
  Type57 : Constant  Value=18
  Type58 : Constant  Value=19
  soc1 : Scope
  Out1 : Outport
  wires:
  Switch2/1 -> Out1/1, soc1/1
  In2/1 -> Sum1/2
  In1/1 -> Sum1/1, Sum/1
  Logical Operator19/1 -> Switch2/2
  Relational Operator3/1 -> Logical Operator19/2
  Type58/1 -> Relational Operator3/2
  Relational Operator2/1 -> Logical Operator19/1
  Type57/1 -> Relational Operator2/2
  Sum/1 -> Switch2/1
  Dot Product2/1 -> Sum/2
  Divide26/1 -> Dot Product2/1
  Type54/1 -> Divide26/2
  Sum1/1 -> Divide26/1
  Clock2/1 -> Sum2/1, Relational Operator2/1, Relational Operator3/1
  Type1/1 -> Sum2/2
  Sum2/1 -> Dot Product2/2

== system Energy_Cost/Battery/Enabled Subsystem1/Subsystem19 ==
  In1 : Inport
  In2 : Inport  Port=2
  Clock2 : Clock
  Divide26 : Product  Inputs=*/
  Dot Product2 : DotProduct  InputSameDT=on  OutDataTypeStr=Inherit: Inherit via internal rule
  Logical Operator19 : Logic  AllPortsSameDT=off  OutDataTypeStr=boolean
  Relational Operator2 : RelationalOperator  RndMeth=Nearest  InputSameDT=on
  Relational Operator3 : RelationalOperator  Operator=<  RndMeth=Nearest  InputSameDT=on
  Sum : Sum  Inputs=|++
  Sum1 : Sum  Inputs=|-+
  Sum2 : Sum  Inputs=|+-
  Switch2 : Switch  Criteria=u2 > Threshold
  Type1 : Constant  Value=19
  Type54 : Constant
  Type57 : Constant  Value=19
  Type58 : Constant  Value=20
  soc1 : Scope
  Out1 : Outport
  wires:
  Sum2/1 -> Dot Product2/2
  Type1/1 -> Sum2/2
  Clock2/1 -> Relational Operator3/1, Relational Operator2/1, Sum2/1
  Sum1/1 -> Divide26/1
  Type54/1 -> Divide26/2
  Divide26/1 -> Dot Product2/1
  Dot Product2/1 -> Sum/2
  Sum/1 -> Switch2/1
  Type57/1 -> Relational Operator2/2
  Relational Operator2/1 -> Logical Operator19/1
  Type58/1 -> Relational Operator3/2
  Relational Operator3/1 -> Logical Operator19/2
  Logical Operator19/1 -> Switch2/2
  In1/1 -> Sum/1, Sum1/1
  In2/1 -> Sum1/2
  Switch2/1 -> soc1/1, Out1/1

== system Energy_Cost/Battery/Enabled Subsystem1/Subsystem2 ==
  In1 : Inport
  In2 : Inport  Port=2
  Clock2 : Clock
  Divide26 : Product  Inputs=*/
  Dot Product2 : DotProduct  InputSameDT=on  OutDataTypeStr=Inherit: Inherit via internal rule
  Logical Operator19 : Logic  AllPortsSameDT=off  OutDataTypeStr=boolean
  Relational Operator2 : RelationalOperator  RndMeth=Nearest  InputSameDT=on
  Relational Operator3 : RelationalOperator  Operator=<  RndMeth=Nearest  InputSameDT=on
  Sum : Sum  Inputs=|++
  Sum1 : Sum  Inputs=|-+
  Sum2 : Sum  Inputs=|+-
  Switch2 : Switch  Criteria=u2 > Threshold
  Type1 : Constant  Value=2
  Type54 : Constant
  Type57 : Constant  Value=2
  Type58 : Constant  Value=3
  soc1 : Scope
  Out1 : Outport
  wires:
  Sum2/1 -> Dot Product2/2
  Type1/1 -> Sum2/2
  Clock2/1 -> Relational Operator3/1, Relational Operator2/1, Sum2/1
  Sum1/1 -> Divide26/1
  Type54/1 -> Divide26/2
  Divide26/1 -> Dot Product2/1
  Dot Product2/1 -> Sum/2
  Sum/1 -> Switch2/1
  Type57/1 -> Relational Operator2/2
  Relational Operator2/1 -> Logical Operator19/1
  Type58/1 -> Relational Operator3/2
  Relational Operator3/1 -> Logical Operator19/2
  Logical Operator19/1 -> Switch2/2
  In1/1 -> Sum/1, Sum1/1
  In2/1 -> Sum1/2
  Switch2/1 -> soc1/1, Out1/1
